simulink model "thermocouple_signal_conditioning"  (R2025a)
settings: Solver=ode45  StartTime=0.0  StopTime=1000  RelTol=1e-3
settings Model: NumberOfSteps=3  Creator=compumarts  LastModifiedBy=compumarts

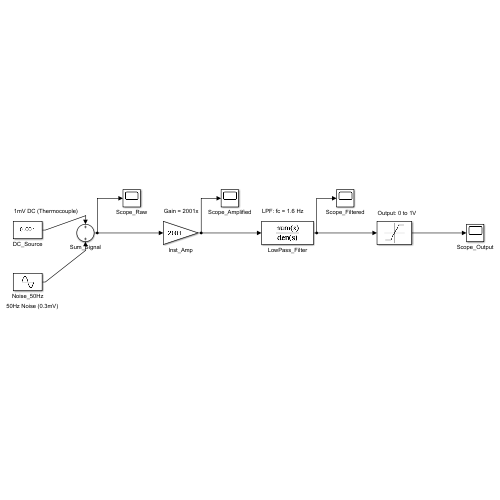
[thumbnail: Simulink's stored preview of the top-level diagram]
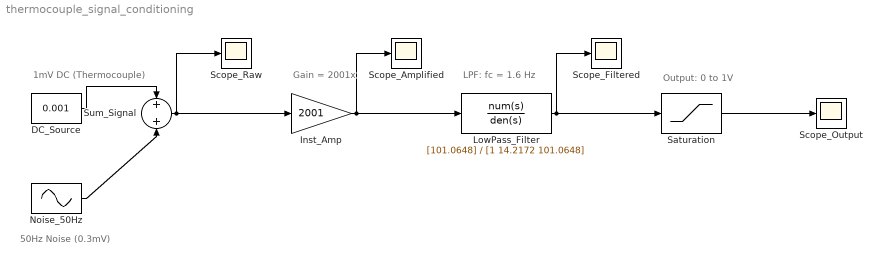
== system thermocouple_signal_conditioning ==
  note: 1mV DC (Thermocouple)
  note: 50Hz Noise (0.3mV)
  note: Gain = 2001x
  note: LPF: fc = 1.6 Hz
  note: Output: 0 to 1V
  DC_Source : Constant  Value=0.001
  Inst_Amp : Gain  Gain=2001
  LowPass_Filter : TransferFcn  Numerator=[101.0648]  Denominator=[1 14.2172 101.0648]
  Noise_50Hz : Sin  Amplitude=0.0003  Frequency=2*pi*50  SampleTime=0
  Saturation : Saturate  UpperLimit=5  LowerLimit=0
  Scope_Amplified : Scope
      settings: ActiveDisplayYMinimum=1.3319672640636249  ActiveDisplayYMaximum=2.6285476405933448
  Scope_Filtered : Scope
      settings: ActiveDisplayYMinimum=-0.26099036235429912  ActiveDisplayYMaximum=2.3489132611886925
  Scope_Output : Scope
      settings: ActiveDisplayYMinimum=-0.26098962729384417  ActiveDisplayYMaximum=2.3489066456445982
  Scope_Raw : Scope
      settings: ActiveDisplayYMinimum=0.00066565080662849278  ActiveDisplayYMaximum=0.0013136170117907776
  Sum_Signal : Sum
  wires:
  DC_Source/1 -> Sum_Signal/1
  Noise_50Hz/1 -> Sum_Signal/2
  Sum_Signal/1 -> Scope_Raw/1, Inst_Amp/1
  Inst_Amp/1 -> Scope_Amplified/1, LowPass_Filter/1
  LowPass_Filter/1 -> Saturation/1, Scope_Filtered/1
  Saturation/1 -> Scope_Output/1
